simulink model "psdcomp"  (R2018b)
settings: Solver=FixedStepDiscrete  StartTime=0.0  StopTime=inf  RelTol=1e-3  AbsTol=1e-6  EnableMultiTasking=on
libraries: dspspect3 x5, dspsrcs4 x1
settings Model: RequirementInfo=9  ExtModeTrigMode=oneshot  ExtModeArmWhenConnect=off  Creator=Wolter  LastModifiedBy=wolter
settings SolverCC: AutoScaleAbsTol=off
settings DataIOCC: SaveFormat=Array  SaveOutput=off  SaveTime=off  SignalLoggingName=sigsOut
settings OptimizationCC: BlockReduction=off  BooleanDataType=off  OptimizeBlockIOStorage=off  BufferReuse=off  GlobalBufferReuse=off  ExpressionFolding=off  ExpressionDepthLimit=2147483647  LocalBlockOutputs=off  RollThreshold=2  InitFltsAndDblsToZero=on  LifeSpan=inf  BufferReusableBoundary=off  OptimizeDataStoreBuffers=off  BusAssignmentInplaceUpdate=off
settings DebuggingCC: SaveWithParameterizedLinksMsg=none  SignalResolutionControl=TryResolveAllWithWarning  MultiTaskDSMMsg=warning  MultiTaskCondExecSysMsg=none  IntegerOverflowMsg=none  BusObjectLabelMismatch=none  StateNameClashWarn=warning  SFUnexpectedBacktrackingDiag=warning  SFNoUnconditionalDefaultTransitionDiag=warning  SFExecutionAtInitializationDiag=none  IntegerSaturationMsg=none
settings HardwareCC: ProdBitPerPointer=32  ProdBitPerSizeT=32  ProdBitPerPtrDiffT=32  ProdLargestAtomicFloat=None  ProdIntDivRoundTo=Undefined  ProdEndianess=Unspecified  ProdWordSize=32  ProdHWDeviceType=Specified
settings ModelReferenceCC: PropagateSignalLabelsOutOfModel=off
settings SFSimCC: SimUseLocalCustomCode=off
settings RTWCC: RTWUseLocalCustomCode=off
settings CodeAppCC: StateflowObjectComments=on
settings GRTTargetCC: TargetFcnLib=ansi_tfl_tmw.mat  TargetLangStandard=C89/C90 (ANSI)  GeneratePreprocessorConditionals=Disable all  CombineOutputUpdateFcns=off  GRTInterface=on
settings ConfigComp: CovMetricSettings=dw  CovHtmlReporting=on  CovSaveCumulativeToWorkspaceVar=on  CovSaveSingleToWorkspaceVar=on  CovExternalEMLEnable=off  CovSFcnEnable=off

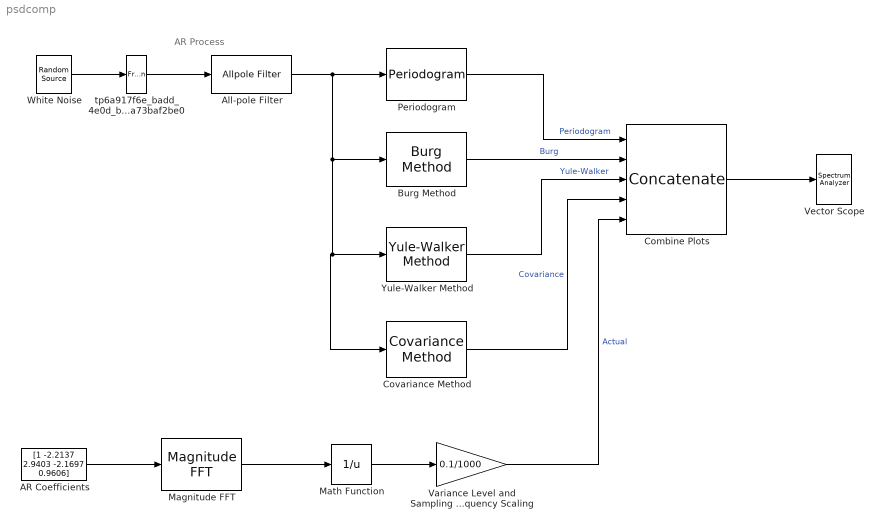
== system psdcomp ==
  note: AR Process
  AR Coefficients : Constant  Value=[1 -2.2137 2.9403 -2.1697 0.9606]
  All-pole Filter : AllpoleFilter  Coefficients=[1 -2.2137 2.9403 -2.1697 0.9606]  AccumDataTypeStr=Inherit: Same as product output
  Burg Method : dspspect3/Burg Method  inheritOrd=off  ord=4  inheritFFT=off  fftsize=128  inheritTs=on  Ts=1
      settings: SourceProductName=DSP System Toolbox  SourceProductBaseCode=DS
  Combine Plots : Concatenate  NumInputs=5  Mode=Multidimensional array  ConcatenateDimension=2
  Covariance Method : dspspect3/Covariance Method  ord=4  inheritFFT=off  fftsize=128  inheritTs=on  Ts=1
      settings: SourceProductName=DSP System Toolbox  SourceProductBaseCode=DS
  Magnitude FFT : dspspect3/Magnitude FFT  mag_or_magsq=Magnitude squared  FFTImplementation=Auto  fftLenInherit=off  fftsize=128  WrapInput=on
      settings: SourceProductName=DSP System Toolbox  SourceProductBaseCode=DS
  Math Function : Math  Operator=reciprocal  SaturateOnIntegerOverflow=on
  Periodogram : dspspect3/Periodogram  measurement=Power spectral density  wintype=Hamming  Rs=50  beta=5  winsamp=Symmetric  FFTImplementation=Auto  inheritFFT=off  fftsize=128  navg=4  inheritTs=on  Ts=1
      settings: SourceProductName=DSP System Toolbox  SourceProductBaseCode=DS
  Variance Level and Sampling Frequency Scaling : Gain  Gain=0.1/1000  SaturateOnIntegerOverflow=on  OutDataTypeStr=Inherit: Same as input  ParamDataTypeStr=Inherit: Same as input
  Vector Scope : SpectrumAnalyzer
  White Noise : dspsrcs4/Random Source  SrcType=Gaussian  NormMethod=Ziggurat  CltLength=12  MinVal=0  MaxVal=1  MeanVal=0  VarVal=0.1  RepMode=Specify seed  rawSeed=0  IsInherit=off  SampMode=Discrete  SampTime=1/1000  SampFrame=64  DataType=Double  OutComplex=Real  OutputFrames=off
  Yule-Walker Method : dspspect3/Yule-Walker Method  inheritOrd=off  ord=6  inheritFFT=off  fftsize=128  inheritTs=on  Ts=1
      settings: SourceProductName=DSP System Toolbox  SourceProductBaseCode=DS
  tp6a917f6e_badd_4e0d_b079_62a73baf2be0 : FrameConversion
  wires:
  Magnitude FFT/1 -> Math Function/1
  AR Coefficients/1 -> Magnitude FFT/1
  All-pole Filter/1 -> Covariance Method/1, Yule-Walker Method/1, Burg Method/1, Periodogram/1
  Math Function/1 -> Variance Level and Sampling Frequency Scaling/1
  Periodogram/1 -> Combine Plots/1  "Periodogram"
  Yule-Walker Method/1 -> Combine Plots/3  "Yule-Walker"
  Burg Method/1 -> Combine Plots/2  "Burg"
  Combine Plots/1 -> Vector Scope/1
  Variance Level and Sampling Frequency Scaling/1 -> Combine Plots/5  "Actual"
  Covariance Method/1 -> Combine Plots/4  "Covariance"
  White Noise/1 -> tp6a917f6e_badd_4e0d_b079_62a73baf2be0/1
  tp6a917f6e_badd_4e0d_b079_62a73baf2be0/1 -> All-pole Filter/1
